simulink model "ladpt"  (Simulink 2.09)
settings: Solver=ode45  StartTime=0.0  StopTime=10.0  RelTol=1e-3  AbsTol=1e-6
undefined symbols (not defined in the file): a, b, c, J, K, k, Mv, p, R, T, U
settings Model: ConsistencyChecking=off  RTWTemplateMakefile=grt_vc.tmf

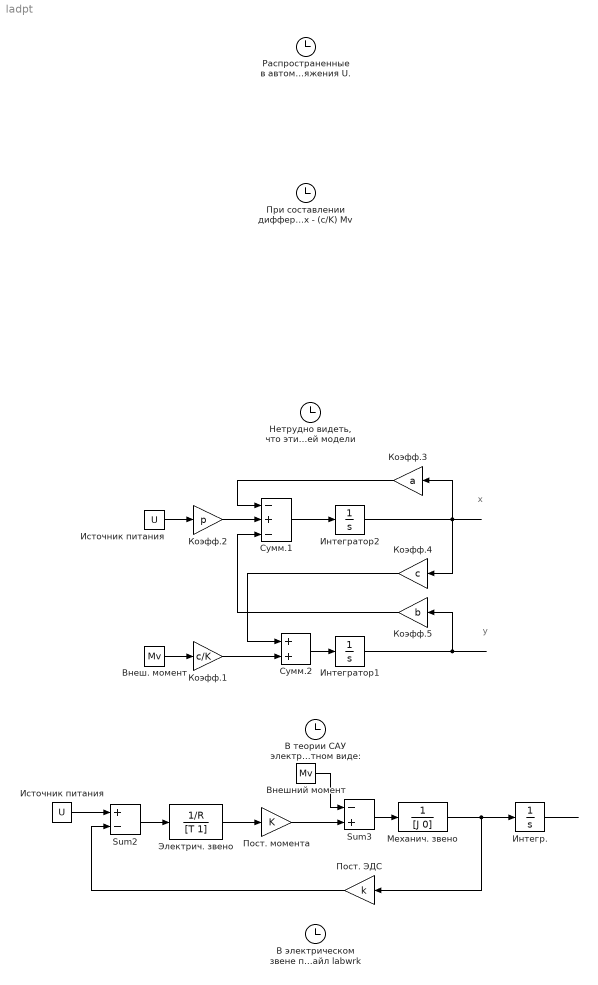
== system ladpt ==
  note: y
  note: x
  Sum2 : Sum  Inputs=+-
  Sum3 : Sum  Inputs=-+
  В теории САУ электроприводом  данную модель принято представлять в эквивалентном виде: : Clock
  "В электрическом звене постоянная времени Т составляет T=R/L. Оконечный интегратор введен для получения значенния угла поворота вала двигателя.  Задание: перерисуйте в отчет данные ( 2) модели. Объясните, как получена вторая модель из первой, в свою очередь полученной непосредственно по уравнениям ДПТ в нормальной форме Коши. Далее закройте данный файл и через главное меню Library: simulink, опцию File откройте файл labwrk" : Clock
  "Внеш. момент         " : Constant  Value=Mv
  "Внешний момент             " : Constant  Value=Mv
  Интегр. : Integrator  ExternalReset=none  InitialConditionSource=internal  InitialCondition=0  LimitOutput=off  UpperSaturationLimit=inf  LowerSaturationLimit=-inf  ShowSaturationPort=off  ShowStatePort=off  AbsoluteTolerance=auto
  Интегратор1 : Integrator  ExternalReset=none  InitialConditionSource=internal  InitialCondition=0  LimitOutput=off  UpperSaturationLimit=inf  LowerSaturationLimit=-inf  ShowSaturationPort=off  ShowStatePort=off  AbsoluteTolerance=auto
  Интегратор2 : Integrator  ExternalReset=none  InitialConditionSource=internal  InitialCondition=0  LimitOutput=off  UpperSaturationLimit=inf  LowerSaturationLimit=-inf  ShowSaturationPort=off  ShowStatePort=off  AbsoluteTolerance=auto
  "Источник питания           " : Constant  Value=U
  "Источник питания                             " : Constant  Value=U
  Коэфф.1 : Gain  Gain=c/K
  "Коэфф.2     " : Gain  Gain=p
  Коэфф.3 : Gain  Orientation=left  Gain=a
  Коэфф.4 : Gain  Orientation=left  Gain=c
  Коэфф.5 : Gain  Orientation=left  Gain=b
  Механич. звено : TransferFcn  Numerator=[1]  Denominator=[J 0]
  "Нетрудно видеть, что эти уравнения приводят к следующей модели" : Clock
  Пост. ЭДС : Gain  Orientation=left  Gain=k
  Пост. момента : Gain  Gain=K
  "При составлении дифференциальных уравнений ДПТ для электрической цепи используется второй закон Кирхгофа, согласно которому: U - E = IR + L( dI/dt ) E = k w            k - коэффициент пропорциональности, называемый постоянной ЭДС двигателя, w - угловая скорость вращения вала двигателя. Составляющая  IR характеризует падение напряжения на активном сопротивлении якорной цепи в соответствии с законом Ома, а L( dI/dt ) отражает наличие ЭДС самоиндукции, возникающей в обмотке при изменении  тока якоря.  Дифференциальное уравнение  механической части двигателя составляется на основании второго закона Ньютона: Md - Mv = J( dw/dt ) Md = K I   Md - момент двигателя,  K - коэффициент пропорциональности,  называемый постоянной момента двигателя,  Mv - момент внешних сил. На основании данных уравнений, вводя обозначения I = x, w = y, 1/L=p, R/L=a, k/L=b, K/J=c, 1/J=c/K, получаем систему дифференциальных  уравнений двигателя в нормальной форме Коши: dx/dt = -ax - by +pU dy/dt = cx - (c/K) Mv " : Clock
  "Распространенные в автоматизированном машиностроении двигатели постоянного тока  (ДПТ)  преобразуют электрическую энергию источника питания, к которому  подключен двигатель, в энергию механического движения ротора и связанного с ним объекта управления.  Принцип работы  ДПТ основан на взаимодействии магнит- ного поля, создаваемого, например, постоянными магнитами, и находящегося в этом поле проводника с током. Математическая модель ДПТ, как динамической сис- темы, может быть построена на базе его достаточных уравнений. В них должны быть учтены как электрическая, так и механическая части двигателя. Электрическая  якорная цепь содержит источник питания с напряжением постоянного тока U, активное сопротивление  R и индуктивность L якорной обмотки,  а также  противоЭДС  двигателя  Е.  Она возникает в соответствии с законами электромагнитной индукции, согласно которым в проводнике , движущимся в магнитном поле,  индуцируется электродвижущая сила (ЭДС). В ДПТ данная ЭДС направлена против внешнего напряжения U." : Clock
  Сумм.1 : Sum  Inputs=-+-
  Сумм.2 : Sum  Inputs=++
  Электрич. звено : TransferFcn  Numerator=1/R  Denominator=[T 1]
  wires:
  "Источник питания           "/1 -> Sum2/1
  Sum2/1 -> Электрич. звено/1
  Электрич. звено/1 -> Пост. момента/1
  Пост. момента/1 -> Sum3/2
  "Внешний момент             "/1 -> Sum3/1
  Механич. звено/1 -> Интегр./1, Пост. ЭДС/1
  Пост. ЭДС/1 -> Sum2/2
  Интегр./1 -> ?
  "Внеш. момент         "/1 -> Коэфф.1/1
  "Источник питания                             "/1 -> "Коэфф.2     "/1
  Интегратор2/1 -> Коэфф.4/1, Коэфф.3/1
  Коэфф.4/1 -> Сумм.2/1
  Коэфф.1/1 -> Сумм.2/2
  Сумм.1/1 -> Интегратор2/1
  Сумм.2/1 -> Интегратор1/1
  Коэфф.5/1 -> Сумм.1/3
  "Коэфф.2     "/1 -> Сумм.1/2
  Коэфф.3/1 -> Сумм.1/1
  Интегратор1/1 -> Коэфф.5/1
  Sum3/1 -> Механич. звено/1
